simulink model "questao7"  (R2023a)
settings: Solver=VariableStepAuto  StartTime=0.0  StopTime=100  RelTol=1e-3
values from neighbouring files (symbols this model uses):
  B = 0.1    [Trab1_real.m]    (also in questao5.m)
  i0 = 0    [Trab1_real.m]    (also in questao5.m)
  J = 1    [Trab1_real.m]    (also in questao5.m)
  K = 1/3    (= 0.333333333333)    [Trab1_real.m]    (also in questao5.m)
  L = 0.5    [Trab1_real.m]    (also in questao5.m)
  R = 10    [Trab1_real.m]    (also in questao5.m)
settings Model: Creator=thiag  LastModifiedBy=thiag

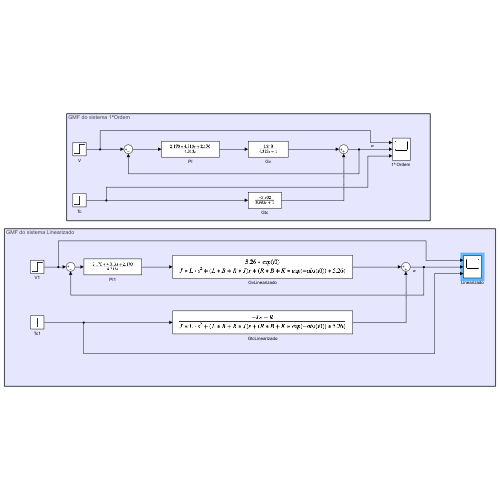
[thumbnail: Simulink's stored preview of the top-level diagram]
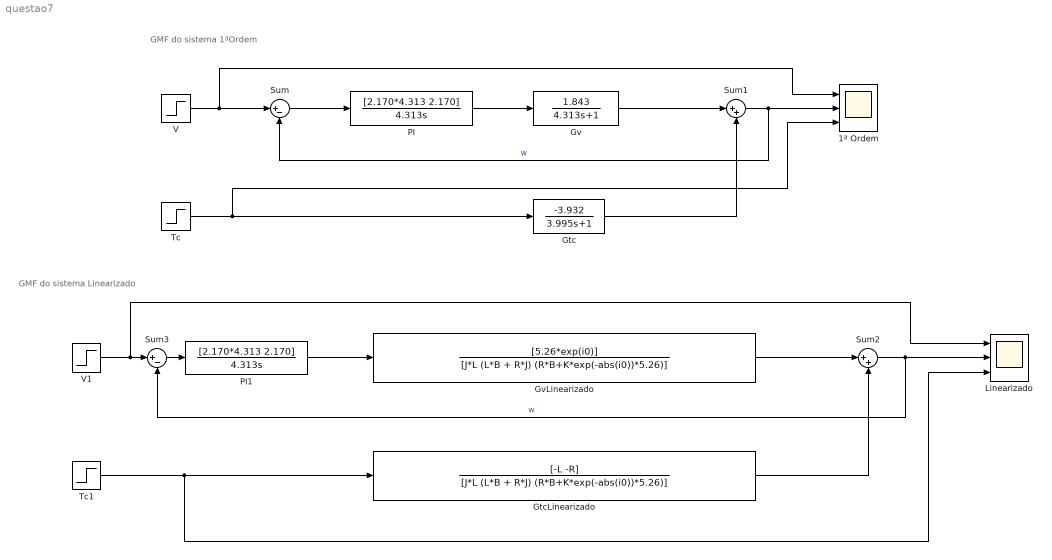
== system questao7 ==
  note: GMF do sistema Linearizado
  note: GMF do sistema 1ªOrdem
  "1ª Ordem " : Scope  NumInputPorts=3
  Gtc : TransferFcn  Numerator=[-3.932]  Denominator=[3.995 1]
  GtcLinearizado : TransferFcn  Numerator=[-L -R]  Denominator=[J*L (L*B + R*J) (R*B+K*exp(-abs(i0))*5.26)]
  Gv : TransferFcn  Numerator=[1.843]  Denominator=[4.313 1]
  GvLinearizado : TransferFcn  Numerator=[5.26*exp(i0)]  Denominator=[J*L (L*B + R*J) (R*B+K*exp(-abs(i0))*5.26)]
  Linearizado : Scope  NumInputPorts=3
  PI : TransferFcn  Numerator=[2.170*4.313 2.170]  Denominator=[4.313 0]
  PI1 : TransferFcn  Numerator=[2.170*4.313 2.170]  Denominator=[4.313 0]
  Sum : Sum  Inputs=|+-
  Sum1 : Sum  Inputs=|++
  Sum2 : Sum  Inputs=|++
  Sum3 : Sum  Inputs=|+-
  Tc : Step  Time=30  After=2  SampleTime=0
  Tc1 : Step  Time=30  After=2  SampleTime=0
  V : Step  Time=10  After=3  SampleTime=0
  V1 : Step  Time=10  After=3  SampleTime=0
  wires:
  V/1 -> "1ª Ordem "/1, Sum/1
  Sum/1 -> PI/1
  PI/1 -> Gv/1
  Gv/1 -> Sum1/1
  Gtc/1 -> Sum1/2
  Tc/1 -> "1ª Ordem "/3, Gtc/1
  Sum1/1 -> Sum/2, "1ª Ordem "/2  "w"
  V1/1 -> Sum3/1, Linearizado/1
  PI1/1 -> GvLinearizado/1
  GvLinearizado/1 -> Sum2/1
  Sum2/1 -> Sum3/2, Linearizado/2  "w"
  GtcLinearizado/1 -> Sum2/2
  Tc1/1 -> Linearizado/3, GtcLinearizado/1
  Sum3/1 -> PI1/1
